simulink model "TestModel_No2"  (R2023b)
settings: Solver=ode45  StartTime=0.0  StopTime=7  FixedStep=0.0104  RelTol=1e-3
InitFcn:
  | Init_TestModel;
StartFcn:
  | Init_TestModel;
undefined symbols (not defined in the file or in its folder): Norm
libraries: slident x1
settings Model: Creator=Selim  LastModifiedBy=Selim

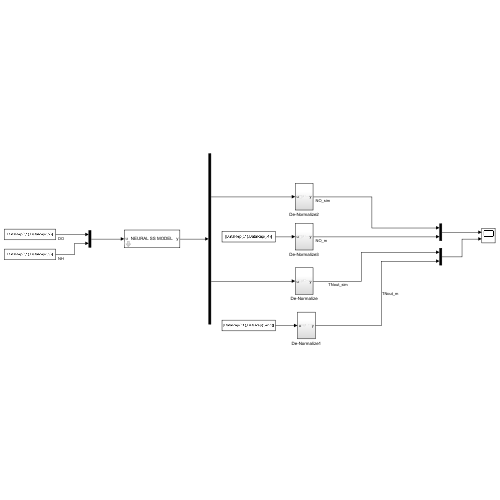
[thumbnail: Simulink's stored preview of the top-level diagram]
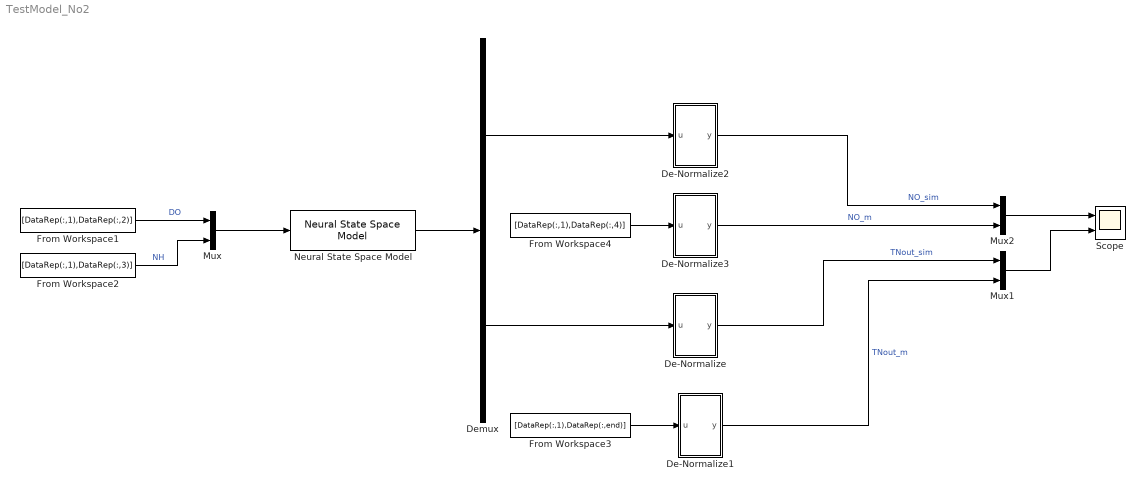
== system TestModel_No2 ==
  De-Normalize : Subsystem
  De-Normalize1 : Subsystem
  De-Normalize2 : Subsystem
  De-Normalize3 : Subsystem
  Demux : Demux  Outputs=2
  From Workspace1 : FromWorkspace  VariableName=[DataRep(:,1),DataRep(:,2)]
  From Workspace2 : FromWorkspace  VariableName=[DataRep(:,1),DataRep(:,3)]
  From Workspace3 : FromWorkspace  VariableName=[DataRep(:,1),DataRep(:,end)]
  From Workspace4 : FromWorkspace  VariableName=[DataRep(:,1),DataRep(:,4)]
  Mux : Mux  Inputs=2
  Mux1 : Mux  Inputs=2
  Mux2 : Mux  Inputs=2
  Neural State Space Model : slident/Models/Neural State Space Model  sys=sys  x0type=internal  ic=[0;0]  returnx=off  returndx=off  domain=CT  feedthroughCT=NoFT  feedthroughDT=FT
  Scope : Scope  NumInputPorts=2
  wires:
  Mux/1 -> Neural State Space Model/1
  Neural State Space Model/1 -> Demux/1
  From Workspace1/1 -> Mux/1  "DO"
  From Workspace2/1 -> Mux/2  "NH"
  De-Normalize/1(y) -> Mux1/1  "TNout_sim"
  From Workspace3/1 -> De-Normalize1/1(u)
  De-Normalize1/1(y) -> Mux1/2  "TNout_m"
  From Workspace4/1 -> De-Normalize3/1(u)
  Demux/1 -> De-Normalize2/1(u)
  Demux/2 -> De-Normalize/1(u)
  De-Normalize3/1(y) -> Mux2/2  "NO_m"
  De-Normalize2/1(y) -> Mux2/1  "NO_sim"
  Mux2/1 -> Scope/1
  Mux1/1 -> Scope/2

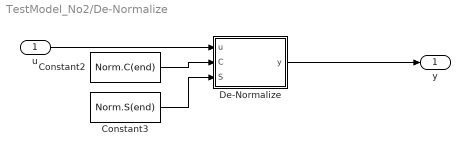
== system TestModel_No2/De-Normalize ==
  u : Inport
  Constant2 : Constant  Value=Norm.C(end)
  Constant3 : Constant  Value=Norm.S(end)
  De-Normalize : MATLAB Function  TreatAsAtomicUnit=on
  y : Outport
  wires:
  Constant2/1 -> De-Normalize/2(C)
  De-Normalize/1(y) -> y/1
  u/1 -> De-Normalize/1(u)
  Constant3/1 -> De-Normalize/3(S)

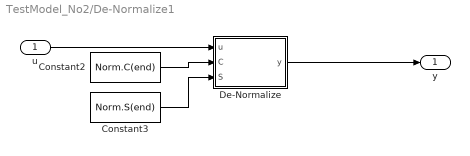
== system TestModel_No2/De-Normalize1 ==
  u : Inport
  Constant2 : Constant  Value=Norm.C(end)
  Constant3 : Constant  Value=Norm.S(end)
  De-Normalize : MATLAB Function  TreatAsAtomicUnit=on
  y : Outport
  wires:
  Constant3/1 -> De-Normalize/3(S)
  u/1 -> De-Normalize/1(u)
  De-Normalize/1(y) -> y/1
  Constant2/1 -> De-Normalize/2(C)

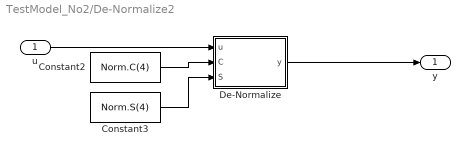
== system TestModel_No2/De-Normalize2 ==
  u : Inport
  Constant2 : Constant  Value=Norm.C(4)
  Constant3 : Constant  Value=Norm.S(4)
  De-Normalize : MATLAB Function  TreatAsAtomicUnit=on
  y : Outport
  wires:
  Constant3/1 -> De-Normalize/3(S)
  u/1 -> De-Normalize/1(u)
  De-Normalize/1(y) -> y/1
  Constant2/1 -> De-Normalize/2(C)

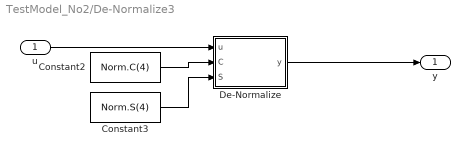
== system TestModel_No2/De-Normalize3 ==
  u : Inport
  Constant2 : Constant  Value=Norm.C(4)
  Constant3 : Constant  Value=Norm.S(4)
  De-Normalize : MATLAB Function  TreatAsAtomicUnit=on
  y : Outport
  wires:
  Constant2/1 -> De-Normalize/2(C)
  De-Normalize/1(y) -> y/1
  u/1 -> De-Normalize/1(u)
  Constant3/1 -> De-Normalize/3(S)

== matlab function TestModel_No2/De-Normalize3/De-Normalize ==
  data: u input; y output; C input; S input
function y = fcn(u,C,S)

y = u * S + C;

end

== matlab function TestModel_No2/De-Normalize/De-Normalize ==
  data: u input; y output; C input; S input
function y = fcn(u,C,S)

y = u * S + C;

end

== matlab function TestModel_No2/De-Normalize1/De-Normalize ==
  data: u input; y output; C input; S input
function y = fcn(u,C,S)

y = u * S + C;

end

== matlab function TestModel_No2/De-Normalize2/De-Normalize ==
  data: u input; y output; C input; S input
function y = fcn(u,C,S)

y = u * S + C;

end
